simulink subsystem "edge1x2_toggleable_asSubsystem"  (R2021a)
settings: Solver=VariableStepAuto  StartTime=0.0  StopTime=10.0  RelTol=1e-3
libraries: EdgesLibrary x2
settings Model: Creator=phill  LastModifiedBy=phill

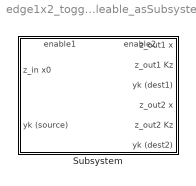
== system edge1x2_toggleable_asSubsystem ==
  Subsystem : Subsystem  mask{tRk=0, w1=0.5}
      mask prompts: tRk "Rk total"; w1 "weight for z_out 1"
      settings: PortSchema="{\"entries\":[{\"content\":{\"sides\":[{\"content\":{\"connectorIds\":[\"In1\",\"Out3\"]},\"type\":\"ConnectorPlacement.EquallySpacedRectSide\",\"uuid\":\"2e9f11d3-65d9-473f-b826-57e0db4d0b8d\"},{\"content\":{\"connectorIds\":[\"In4\",\"In5\",\"Out1\",\"In6\",\"In7\",\"Out2\"],\"side\":\"RIGHT\"},\"type\":\"ConnectorPlacement.EquallySpacedRectSide\",\"uuid\":\"d8eabf6d-fb3a-4c3e-97ce-4f99fedc7242\"},{\"content\":{\"connectorIds\":[\"In2\",\"In3\"],\"side\":\"TOP\"},\"type\":\"ConnectorPlacement.EquallySpacedRectSide\",\"uuid\":\"c1317a9d-7aa4-490c-a27e-f3fa93a0d151\"}]},\"type\":\"ConnectorPlacement.EquallySpacedConnector\",\"uuid\":\"3cd892e4-da09-4624-b831-53c46896b420\"}],\"packageUris\":[\"http://schema.mathworks.com/mf0/Connector/R2020b\"],\"version\":\"1.0\"}"
      mask Display:
      | image('$imagefile'); % Use "Edit Image" on toolstrip to change.
      | disp('Toggleable Edge 1x2 \n\n');
      | tRk = get_param(gcb,'tRk');
      | w1 = get_param(gcb, 'w1');
      | disp(['Rk = ', tRk, ' | w1 =  ', w1])

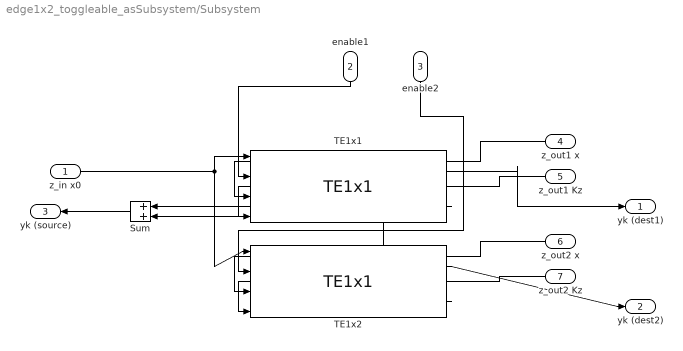
== system edge1x2_toggleable_asSubsystem/Subsystem ==
  z_in x0 : Inport
  enable1 : Inport  Port=2
  enable2 : Inport  Port=3
  z_out1 x : Inport  Port=4
  z_out1 Kz : Inport  Port=5
  z_out2 x : Inport  Port=6
  z_out2 Kz : Inport  Port=7
  Sum : Sum
  TE1x1 : EdgesLibrary/TE1x1  Rk=w1*tRk
  TE1x2 : EdgesLibrary/TE1x1  Rk=(1-w1)*tRk
  yk (dest1) : Outport
  yk (dest2) : Outport  Port=2
  yk (source) : Outport  Port=3
  wires:
  TE1x1/1 -> yk (dest1)/1
  enable1/1 -> TE1x1/2
  z_out1 x/1 -> TE1x1/3
  z_out1 Kz/1 -> TE1x1/4
  TE1x2/1 -> yk (dest2)/1
  TE1x2/2 -> Sum/2
  z_out2 Kz/1 -> TE1x2/4
  z_in x0/1 -> TE1x2/1, TE1x1/1
  TE1x1/2 -> Sum/1
  Sum/1 -> yk (source)/1
  z_out2 x/1 -> TE1x2/3
  enable2/1 -> TE1x2/2
